simulink model "Model_Simulation"  (R2016a)
settings: Solver=FixedStepAuto  StartTime=0.0  StopTime=5  FixedStep=2e-6  RelTol=1e-3
values from neighbouring files (symbols this model uses):
  C = 3060e-6    (= 0.00306)    [Controle_Inversor_UR_D.m]
  Ki_i_disc = wc*Rf    (= 44.2477838534)    [Controle_Inversor_UR_D.m]
  Ki_i_disc_b = wc_b*Rb/Vdc    (= 0.0983284085631)    [Controle_Inversor_UR_D.m]
  Ki_q_disc = wq/H    [Controle_Inversor_UR_D.m]
  Ki_v_disc_b = wc_bv/Req    (= 14.5799013102)    [Controle_Inversor_UR_D.m]
  Ki_vdc_disc = ((wvdc)^2*C)/Gt    [Controle_Inversor_UR_D.m]
  Kp_i_disc = wc*Lf    (= 2.19688771906)    [Controle_Inversor_UR_D.m]
  Kp_i_disc_b = wc_b*Lb/Vdc    (= 0.00545604673435)    [Controle_Inversor_UR_D.m]
  Kp_q_disc = Ki_q_disc*(Lf/Kp_i_disc)    [Controle_Inversor_UR_D.m]
  Kp_v_disc_b = wc_bv*Cin    (= 0.0356301510224)    [Controle_Inversor_UR_D.m]
  Kp_vdc_disc = (2*ksi_vdc*wvdc*C)/Gt    [Controle_Inversor_UR_D.m]
  Lf = (0.0012+2.8949e-04)    (= 0.00148949)    [Controle_Inversor_UR_D.m]
  Tsw = 1/fsw    (= 0.0002)    [Controle_Inversor_UR_D.m]
  w = 2*pi*60    (= 376.991118431)    [Controle_Inversor_UR_D.m]
undefined symbols (not defined in the file or in its folder): D1, dEgdT, Delta, EgRef, gcbh, k1, Rsh_array5pc, sigbuilder_block, sps_rtmsupport, Tref_K, VT_ref
libraries: powerlib x179, simulink x14, powerlib_meascontrol x13, spsPVarrayModel x12
(part 19 of 20)

== system Model_Simulation/Subsystem2/DDSRF-PLL  ==
  Vabc : Inport
  Constant : Constant  Value=2*pi*60
  Demux : Demux  Outputs=3
  Função transferência LPF Fc = 42 Hz{,1..3} (4 alike) : TransferFcn  Numerator=[0 0 263.8937]  Denominator=[0 1 263.8937]
  Integrator : Integrator
  PID Controller : simulink/Continuous/PID Controller  Controller=PI  TimeDomain=Continuous-time  SampleTime=-1  IntegratorMethod=Forward Euler  FilterMethod=Forward Euler  Form=Parallel  UseFilter=on  ControllerParametersSource=internal  P=0.34  I=38.3  D=0  N=100  InitialConditionSource=internal  InitialConditionForIntegrator=0  InitialConditionForFilter=0  ExternalReset=none  LimitOutput=off  UpperSaturationLimit=inf  LowerSaturationLimit=-inf  LinearizeAsGain=on  AntiWindupMode=none  Kb=1  TrackingMode=off  Kt=1  PParamMin=[]  PParamMax=[]  IParamMin=[]  IParamMax=[]  DParamMin=[]  DParamMax=[]  NParamMin=[]  NParamMax=[]  KbParamMin=[]  KbParamMax=[]  KtParamMin=[]  KtParamMax=[]  POutMin=[]  POutMax=[]  IOutMin=[]  IOutMax=[]  DOutMin=[]  DOutMax=[]  NOutMin=[]  NOutMax=[]  KbOutMin=[]  KbOutMax=[]  KtOutMin=[]  KtOutMax=[]  IntegratorOutMin=[]  IntegratorOutMax=[]  FilterOutMin=[]  FilterOutMax=[]  SumOutMin=[]  SumOutMax=[]  SumI1OutMin=[]  SumI1OutMax=[]  SumI2OutMin=[]  SumI2OutMax=[]  SumI3OutMin=[]  SumI3OutMax=[]  SumDOutMin=[]  SumDOutMax=[]  SaturationOutMin=[]  SaturationOutMax=[]  IntegratorContinuousStateAttributes=''  IntegratorStateMustResolveToSignalObject=off  IntegratorRTWStateStorageClass=Auto  FilterContinuousStateAttributes=''  FilterStateMustResolveToSignalObject=off  FilterRTWStateStorageClass=Auto  DifferentiatorICPrevScaledInput=0  DifferentiatorOutMin=[]  DifferentiatorOutMax=[]
  Subsystem : Subsystem
  Subsystem1 : Subsystem
  Subsystem2 : Subsystem
  Subsystem3 : Subsystem
  Sum : Sum  Inputs=|++
  abc to Alpha-Beta-Zero1 : powerlib_meascontrol/Transformations/abc to Alpha-Beta-Zero
  wt : Outport
  wires:
  Vabc/1 -> abc to Alpha-Beta-Zero1/1
  abc to Alpha-Beta-Zero1/1 -> Demux/1
  Demux/1 -> Subsystem1/2(Alpha), Subsystem/2(Alpha)
  Demux/2 -> Subsystem1/3(Beta), Subsystem/3(Beta)
  Subsystem/1(Vd+) -> Subsystem2/1(Vd+)
  Subsystem/2(Vq+) -> Subsystem2/2(Vq+)
  Subsystem1/1(Vd-) -> Subsystem3/1(Vd-)
  Subsystem1/2(Vq-) -> Subsystem3/2(Vq-)
  Subsystem2/1(Vd*+) -> Função transferência LPF Fc = 42 Hz/1
  Subsystem3/1(Vd*-) -> Função transferência LPF Fc = 42 Hz2/1
  Subsystem3/2(Vq*-) -> Função transferência LPF Fc = 42 Hz3/1
  Função transferência LPF Fc = 42 Hz2/1 -> Subsystem2/3(Vd-)
  Função transferência LPF Fc = 42 Hz3/1 -> Subsystem2/4(Vq-)
  Subsystem2/2(Vq*+) -> PID Controller/1, Função transferência LPF Fc = 42 Hz1/1
  PID Controller/1 -> Sum/1
  Constant/1 -> Sum/2
  Sum/1 -> Integrator/1
  Integrator/1 -> Subsystem2/5(fase), Subsystem3/5(fase), Subsystem1/1(Fase), Subsystem/1(Fase), wt/1
  Função transferência LPF Fc = 42 Hz1/1 -> Subsystem3/4(Vq+)
  Função transferência LPF Fc = 42 Hz/1 -> Subsystem3/3(Vd+)

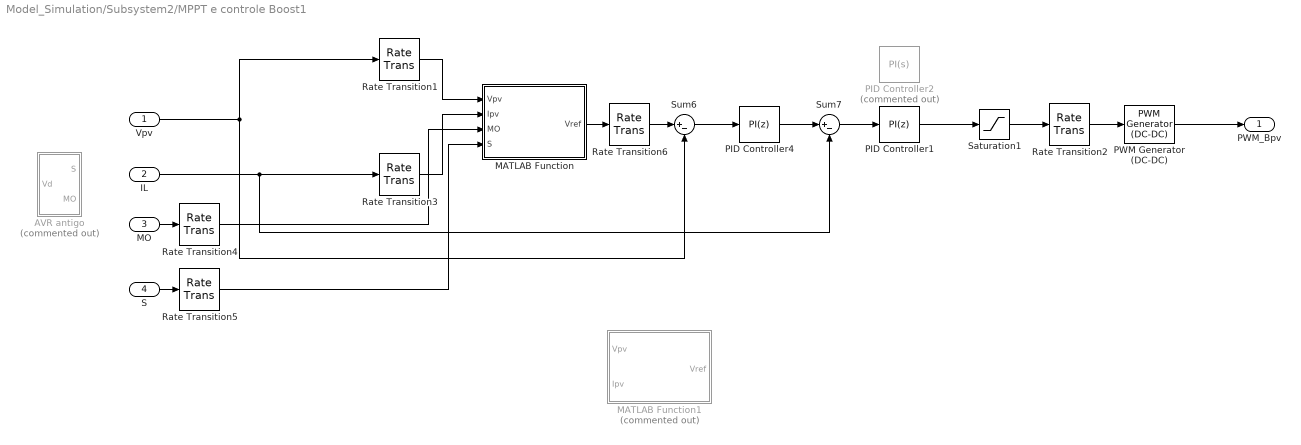
== system Model_Simulation/Subsystem2/MPPT e controle Boost1 ==
  Vpv : Inport
  IL : Inport  Port=2
  MO : Inport  Port=3
  S : Inport  Port=4
  AVR antigo : Subsystem  Commented=on
  MATLAB Function : MATLAB Function  TreatAsAtomicUnit=on
  MATLAB Function1 : MATLAB Function  Commented=on  TreatAsAtomicUnit=on
  PID Controller1 : simulink/Continuous/PID Controller  Controller=PI  TimeDomain=Discrete-time  SampleTime=-1  IntegratorMethod=Trapezoidal  FilterMethod=Forward Euler  Form=Parallel  UseFilter=on  ControllerParametersSource=internal  P=Kp_i_disc_b  I=Ki_i_disc_b  D=0  N=100  InitialConditionSource=internal  InitialConditionForIntegrator=0  InitialConditionForFilter=0  ExternalReset=none  LimitOutput=off  UpperSaturationLimit=inf  LowerSaturationLimit=-inf  LinearizeAsGain=on  AntiWindupMode=none  Kb=1  TrackingMode=off  Kt=1  PParamMin=[]  PParamMax=[]  IParamMin=[]  IParamMax=[]  DParamMin=[]  DParamMax=[]  NParamMin=[]  NParamMax=[]  KbParamMin=[]  KbParamMax=[]  KtParamMin=[]  KtParamMax=[]  POutMin=[]  POutMax=[]  IOutMin=[]  IOutMax=[]  DOutMin=[]  DOutMax=[]  NOutMin=[]  NOutMax=[]  KbOutMin=[]  KbOutMax=[]  KtOutMin=[]  KtOutMax=[]  IntegratorOutMin=[]  IntegratorOutMax=[]  FilterOutMin=[]  FilterOutMax=[]  SumOutMin=[]  SumOutMax=[]  SumI1OutMin=[]  SumI1OutMax=[]  SumI2OutMin=[]  SumI2OutMax=[]  SumI3OutMin=[]  SumI3OutMax=[]  SumDOutMin=[]  SumDOutMax=[]  SaturationOutMin=[]  SaturationOutMax=[]  IntegratorContinuousStateAttributes=''  IntegratorStateMustResolveToSignalObject=off  IntegratorRTWStateStorageClass=Auto  FilterContinuousStateAttributes=''  FilterStateMustResolveToSignalObject=off  FilterRTWStateStorageClass=Auto  DifferentiatorICPrevScaledInput=0  DifferentiatorOutMin=[]  DifferentiatorOutMax=[]
  PID Controller2 : simulink/Continuous/PID Controller  Commented=on  Controller=PI  TimeDomain=Continuous-time  SampleTime=-1  IntegratorMethod=Forward Euler  FilterMethod=Forward Euler  Form=Parallel  UseFilter=on  ControllerParametersSource=internal  P=0.00831222  I=15.393  D=0  N=100  InitialConditionSource=internal  InitialConditionForIntegrator=0  InitialConditionForFilter=0  ExternalReset=none  LimitOutput=off  UpperSaturationLimit=inf  LowerSaturationLimit=-inf  LinearizeAsGain=on  AntiWindupMode=none  Kb=1  TrackingMode=off  Kt=1  PParamMin=[]  PParamMax=[]  IParamMin=[]  IParamMax=[]  DParamMin=[]  DParamMax=[]  NParamMin=[]  NParamMax=[]  KbParamMin=[]  KbParamMax=[]  KtParamMin=[]  KtParamMax=[]  POutMin=[]  POutMax=[]  IOutMin=[]  IOutMax=[]  DOutMin=[]  DOutMax=[]  NOutMin=[]  NOutMax=[]  KbOutMin=[]  KbOutMax=[]  KtOutMin=[]  KtOutMax=[]  IntegratorOutMin=[]  IntegratorOutMax=[]  FilterOutMin=[]  FilterOutMax=[]  SumOutMin=[]  SumOutMax=[]  SumI1OutMin=[]  SumI1OutMax=[]  SumI2OutMin=[]  SumI2OutMax=[]  SumI3OutMin=[]  SumI3OutMax=[]  SumDOutMin=[]  SumDOutMax=[]  SaturationOutMin=[]  SaturationOutMax=[]  IntegratorContinuousStateAttributes=''  IntegratorStateMustResolveToSignalObject=off  IntegratorRTWStateStorageClass=Auto  FilterContinuousStateAttributes=''  FilterStateMustResolveToSignalObject=off  FilterRTWStateStorageClass=Auto  DifferentiatorICPrevScaledInput=0  DifferentiatorOutMin=[]  DifferentiatorOutMax=[]
  PID Controller4 : simulink/Continuous/PID Controller  Controller=PI  TimeDomain=Discrete-time  SampleTime=-1  IntegratorMethod=Trapezoidal  FilterMethod=Forward Euler  Form=Parallel  UseFilter=on  ControllerParametersSource=internal  P=-Kp_v_disc_b  I=-Ki_v_disc_b  D=0  N=100  InitialConditionSource=internal  InitialConditionForIntegrator=0  InitialConditionForFilter=0  ExternalReset=none  LimitOutput=off  UpperSaturationLimit=inf  LowerSaturationLimit=-inf  LinearizeAsGain=on  AntiWindupMode=none  Kb=1  TrackingMode=off  Kt=1  PParamMin=[]  PParamMax=[]  IParamMin=[]  IParamMax=[]  DParamMin=[]  DParamMax=[]  NParamMin=[]  NParamMax=[]  KbParamMin=[]  KbParamMax=[]  KtParamMin=[]  KtParamMax=[]  POutMin=[]  POutMax=[]  IOutMin=[]  IOutMax=[]  DOutMin=[]  DOutMax=[]  NOutMin=[]  NOutMax=[]  KbOutMin=[]  KbOutMax=[]  KtOutMin=[]  KtOutMax=[]  IntegratorOutMin=[]  IntegratorOutMax=[]  FilterOutMin=[]  FilterOutMax=[]  SumOutMin=[]  SumOutMax=[]  SumI1OutMin=[]  SumI1OutMax=[]  SumI2OutMin=[]  SumI2OutMax=[]  SumI3OutMin=[]  SumI3OutMax=[]  SumDOutMin=[]  SumDOutMax=[]  SaturationOutMin=[]  SaturationOutMax=[]  IntegratorContinuousStateAttributes=''  IntegratorStateMustResolveToSignalObject=off  IntegratorRTWStateStorageClass=Auto  FilterContinuousStateAttributes=''  FilterStateMustResolveToSignalObject=off  FilterRTWStateStorageClass=Auto  DifferentiatorICPrevScaledInput=0  DifferentiatorOutMin=[]  DifferentiatorOutMax=[]
  PWM Generator (DC-DC) : powerlib_meascontrol/Pulse & Signal Generators/PWM Generator (DC-DC)  Fsw=5e3  Ts=2e-6
  Rate Transition{1,3..5} (4 alike) : RateTransition  OutPortSampleTime=0.01
  Rate Transition2 : RateTransition  OutPortSampleTime=2e-6
  Rate Transition6 : RateTransition  OutPortSampleTime=Tsw
  Saturation1 : Saturate  UpperLimit=1  LowerLimit=0.01
  Sum6 : Sum  Inputs=|+-
  Sum7 : Sum  Inputs=|+-
  PWM_Bpv : Outport
  wires:
  PID Controller4/1 -> Sum7/1
  Sum6/1 -> PID Controller4/1
  PWM Generator (DC-DC)/1 -> PWM_Bpv/1
  Sum7/1 -> PID Controller1/1
  PID Controller1/1 -> Saturation1/1
  Saturation1/1 -> Rate Transition2/1
  MATLAB Function/1(Vref) -> Rate Transition6/1
  Vpv/1 -> Rate Transition1/1, Sum6/2
  IL/1 -> Rate Transition3/1, Sum7/2
  MO/1 -> Rate Transition4/1
  S/1 -> Rate Transition5/1
  Rate Transition2/1 -> PWM Generator (DC-DC)/1
  Rate Transition1/1 -> MATLAB Function/1(Vpv)
  Rate Transition3/1 -> MATLAB Function/2(Ipv)
  Rate Transition4/1 -> MATLAB Function/3(MO)
  Rate Transition5/1 -> MATLAB Function/4(S)
  Rate Transition6/1 -> Sum6/1

== system Model_Simulation/Subsystem2/MPPT e controle Boost2 ==
  Vpv : Inport
  IL : Inport  Port=2
  MO : Inport  Port=3
  S : Inport  Port=4
  MATLAB Function : MATLAB Function  TreatAsAtomicUnit=on
  MATLAB Function1 : MATLAB Function  Commented=on  TreatAsAtomicUnit=on
  PID Controller1 : simulink/Continuous/PID Controller  Controller=PI  TimeDomain=Discrete-time  SampleTime=-1  IntegratorMethod=Trapezoidal  FilterMethod=Forward Euler  Form=Parallel  UseFilter=on  ControllerParametersSource=internal  P=Kp_i_disc_b  I=Ki_i_disc_b  D=0  N=100  InitialConditionSource=internal  InitialConditionForIntegrator=0  InitialConditionForFilter=0  ExternalReset=none  LimitOutput=off  UpperSaturationLimit=inf  LowerSaturationLimit=-inf  LinearizeAsGain=on  AntiWindupMode=none  Kb=1  TrackingMode=off  Kt=1  PParamMin=[]  PParamMax=[]  IParamMin=[]  IParamMax=[]  DParamMin=[]  DParamMax=[]  NParamMin=[]  NParamMax=[]  KbParamMin=[]  KbParamMax=[]  KtParamMin=[]  KtParamMax=[]  POutMin=[]  POutMax=[]  IOutMin=[]  IOutMax=[]  DOutMin=[]  DOutMax=[]  NOutMin=[]  NOutMax=[]  KbOutMin=[]  KbOutMax=[]  KtOutMin=[]  KtOutMax=[]  IntegratorOutMin=[]  IntegratorOutMax=[]  FilterOutMin=[]  FilterOutMax=[]  SumOutMin=[]  SumOutMax=[]  SumI1OutMin=[]  SumI1OutMax=[]  SumI2OutMin=[]  SumI2OutMax=[]  SumI3OutMin=[]  SumI3OutMax=[]  SumDOutMin=[]  SumDOutMax=[]  SaturationOutMin=[]  SaturationOutMax=[]  IntegratorContinuousStateAttributes=''  IntegratorStateMustResolveToSignalObject=off  IntegratorRTWStateStorageClass=Auto  FilterContinuousStateAttributes=''  FilterStateMustResolveToSignalObject=off  FilterRTWStateStorageClass=Auto  DifferentiatorICPrevScaledInput=0  DifferentiatorOutMin=[]  DifferentiatorOutMax=[]
  PID Controller2 : simulink/Continuous/PID Controller  Commented=on  Controller=PI  TimeDomain=Continuous-time  SampleTime=-1  IntegratorMethod=Forward Euler  FilterMethod=Forward Euler  Form=Parallel  UseFilter=on  ControllerParametersSource=internal  P=-0.02947505  I=-5.3591  D=0  N=100  InitialConditionSource=internal  InitialConditionForIntegrator=0  InitialConditionForFilter=0  ExternalReset=none  LimitOutput=off  UpperSaturationLimit=inf  LowerSaturationLimit=-inf  LinearizeAsGain=on  AntiWindupMode=none  Kb=1  TrackingMode=off  Kt=1  PParamMin=[]  PParamMax=[]  IParamMin=[]  IParamMax=[]  DParamMin=[]  DParamMax=[]  NParamMin=[]  NParamMax=[]  KbParamMin=[]  KbParamMax=[]  KtParamMin=[]  KtParamMax=[]  POutMin=[]  POutMax=[]  IOutMin=[]  IOutMax=[]  DOutMin=[]  DOutMax=[]  NOutMin=[]  NOutMax=[]  KbOutMin=[]  KbOutMax=[]  KtOutMin=[]  KtOutMax=[]  IntegratorOutMin=[]  IntegratorOutMax=[]  FilterOutMin=[]  FilterOutMax=[]  SumOutMin=[]  SumOutMax=[]  SumI1OutMin=[]  SumI1OutMax=[]  SumI2OutMin=[]  SumI2OutMax=[]  SumI3OutMin=[]  SumI3OutMax=[]  SumDOutMin=[]  SumDOutMax=[]  SaturationOutMin=[]  SaturationOutMax=[]  IntegratorContinuousStateAttributes=''  IntegratorStateMustResolveToSignalObject=off  IntegratorRTWStateStorageClass=Auto  FilterContinuousStateAttributes=''  FilterStateMustResolveToSignalObject=off  FilterRTWStateStorageClass=Auto  DifferentiatorICPrevScaledInput=0  DifferentiatorOutMin=[]  DifferentiatorOutMax=[]
  PID Controller4 : simulink/Continuous/PID Controller  Controller=PI  TimeDomain=Discrete-time  SampleTime=-1  IntegratorMethod=Trapezoidal  FilterMethod=Forward Euler  Form=Parallel  UseFilter=on  ControllerParametersSource=internal  P=-Kp_v_disc_b  I=-Ki_v_disc_b  D=0  N=100  InitialConditionSource=internal  InitialConditionForIntegrator=0  InitialConditionForFilter=0  ExternalReset=none  LimitOutput=off  UpperSaturationLimit=inf  LowerSaturationLimit=-inf  LinearizeAsGain=on  AntiWindupMode=none  Kb=1  TrackingMode=off  Kt=1  PParamMin=[]  PParamMax=[]  IParamMin=[]  IParamMax=[]  DParamMin=[]  DParamMax=[]  NParamMin=[]  NParamMax=[]  KbParamMin=[]  KbParamMax=[]  KtParamMin=[]  KtParamMax=[]  POutMin=[]  POutMax=[]  IOutMin=[]  IOutMax=[]  DOutMin=[]  DOutMax=[]  NOutMin=[]  NOutMax=[]  KbOutMin=[]  KbOutMax=[]  KtOutMin=[]  KtOutMax=[]  IntegratorOutMin=[]  IntegratorOutMax=[]  FilterOutMin=[]  FilterOutMax=[]  SumOutMin=[]  SumOutMax=[]  SumI1OutMin=[]  SumI1OutMax=[]  SumI2OutMin=[]  SumI2OutMax=[]  SumI3OutMin=[]  SumI3OutMax=[]  SumDOutMin=[]  SumDOutMax=[]  SaturationOutMin=[]  SaturationOutMax=[]  IntegratorContinuousStateAttributes=''  IntegratorStateMustResolveToSignalObject=off  IntegratorRTWStateStorageClass=Auto  FilterContinuousStateAttributes=''  FilterStateMustResolveToSignalObject=off  FilterRTWStateStorageClass=Auto  DifferentiatorICPrevScaledInput=0  DifferentiatorOutMin=[]  DifferentiatorOutMax=[]
  PWM Generator (DC-DC) : powerlib_meascontrol/Pulse & Signal Generators/PWM Generator (DC-DC)  Fsw=5e3  Ts=2e-6
  Rate Transition{1,3..5} (4 alike) : RateTransition  OutPortSampleTime=0.01
  Rate Transition2 : RateTransition  OutPortSampleTime=2e-6
  Rate Transition6 : RateTransition  OutPortSampleTime=Tsw
  Saturation1 : Saturate  UpperLimit=1  LowerLimit=0.01
  Sum6 : Sum  Inputs=|+-
  Sum7 : Sum  Inputs=|+-
  PWM_Bpv : Outport
  wires:
  IL/1 -> Rate Transition3/1, Sum7/2
  Vpv/1 -> Rate Transition1/1, Sum6/2
  MATLAB Function/1(Vref) -> Rate Transition6/1
  Saturation1/1 -> Rate Transition2/1
  PID Controller1/1 -> Saturation1/1
  Sum7/1 -> PID Controller1/1
  PWM Generator (DC-DC)/1 -> PWM_Bpv/1
  Sum6/1 -> PID Controller4/1
  PID Controller4/1 -> Sum7/1
  MO/1 -> Rate Transition5/1
  S/1 -> Rate Transition4/1
  Rate Transition2/1 -> PWM Generator (DC-DC)/1
  Rate Transition1/1 -> MATLAB Function/1(Vpv)
  Rate Transition3/1 -> MATLAB Function/2(Ipv)
  Rate Transition4/1 -> MATLAB Function/4(S)
  Rate Transition5/1 -> MATLAB Function/3(MO)
  Rate Transition6/1 -> Sum6/1

== system Model_Simulation/Subsystem2/MPPT e controle Boost3 ==
  Vpv : Inport
  IL : Inport  Port=2
  MO : Inport  Port=3
  S : Inport  Port=4
  MATLAB Function : MATLAB Function  TreatAsAtomicUnit=on
  PID Controller1 : simulink/Continuous/PID Controller  Controller=PI  TimeDomain=Discrete-time  SampleTime=-1  IntegratorMethod=Trapezoidal  FilterMethod=Forward Euler  Form=Parallel  UseFilter=on  ControllerParametersSource=internal  P=Kp_i_disc_b  I=Ki_i_disc_b  D=0  N=100  InitialConditionSource=internal  InitialConditionForIntegrator=0  InitialConditionForFilter=0  ExternalReset=none  LimitOutput=off  UpperSaturationLimit=inf  LowerSaturationLimit=-inf  LinearizeAsGain=on  AntiWindupMode=none  Kb=1  TrackingMode=off  Kt=1  PParamMin=[]  PParamMax=[]  IParamMin=[]  IParamMax=[]  DParamMin=[]  DParamMax=[]  NParamMin=[]  NParamMax=[]  KbParamMin=[]  KbParamMax=[]  KtParamMin=[]  KtParamMax=[]  POutMin=[]  POutMax=[]  IOutMin=[]  IOutMax=[]  DOutMin=[]  DOutMax=[]  NOutMin=[]  NOutMax=[]  KbOutMin=[]  KbOutMax=[]  KtOutMin=[]  KtOutMax=[]  IntegratorOutMin=[]  IntegratorOutMax=[]  FilterOutMin=[]  FilterOutMax=[]  SumOutMin=[]  SumOutMax=[]  SumI1OutMin=[]  SumI1OutMax=[]  SumI2OutMin=[]  SumI2OutMax=[]  SumI3OutMin=[]  SumI3OutMax=[]  SumDOutMin=[]  SumDOutMax=[]  SaturationOutMin=[]  SaturationOutMax=[]  IntegratorContinuousStateAttributes=''  IntegratorStateMustResolveToSignalObject=off  IntegratorRTWStateStorageClass=Auto  FilterContinuousStateAttributes=''  FilterStateMustResolveToSignalObject=off  FilterRTWStateStorageClass=Auto  DifferentiatorICPrevScaledInput=0  DifferentiatorOutMin=[]  DifferentiatorOutMax=[]
  PID Controller4 : simulink/Continuous/PID Controller  Controller=PI  TimeDomain=Discrete-time  SampleTime=-1  IntegratorMethod=Trapezoidal  FilterMethod=Forward Euler  Form=Parallel  UseFilter=on  ControllerParametersSource=internal  P=-Kp_v_disc_b  I=-Ki_v_disc_b  D=0  N=100  InitialConditionSource=internal  InitialConditionForIntegrator=0  InitialConditionForFilter=0  ExternalReset=none  LimitOutput=off  UpperSaturationLimit=inf  LowerSaturationLimit=-inf  LinearizeAsGain=on  AntiWindupMode=none  Kb=1  TrackingMode=off  Kt=1  PParamMin=[]  PParamMax=[]  IParamMin=[]  IParamMax=[]  DParamMin=[]  DParamMax=[]  NParamMin=[]  NParamMax=[]  KbParamMin=[]  KbParamMax=[]  KtParamMin=[]  KtParamMax=[]  POutMin=[]  POutMax=[]  IOutMin=[]  IOutMax=[]  DOutMin=[]  DOutMax=[]  NOutMin=[]  NOutMax=[]  KbOutMin=[]  KbOutMax=[]  KtOutMin=[]  KtOutMax=[]  IntegratorOutMin=[]  IntegratorOutMax=[]  FilterOutMin=[]  FilterOutMax=[]  SumOutMin=[]  SumOutMax=[]  SumI1OutMin=[]  SumI1OutMax=[]  SumI2OutMin=[]  SumI2OutMax=[]  SumI3OutMin=[]  SumI3OutMax=[]  SumDOutMin=[]  SumDOutMax=[]  SaturationOutMin=[]  SaturationOutMax=[]  IntegratorContinuousStateAttributes=''  IntegratorStateMustResolveToSignalObject=off  IntegratorRTWStateStorageClass=Auto  FilterContinuousStateAttributes=''  FilterStateMustResolveToSignalObject=off  FilterRTWStateStorageClass=Auto  DifferentiatorICPrevScaledInput=0  DifferentiatorOutMin=[]  DifferentiatorOutMax=[]
  PWM Generator (DC-DC) : powerlib_meascontrol/Pulse & Signal Generators/PWM Generator (DC-DC)  Fsw=5e3  Ts=2e-6
  Rate Transition{1,3..5} (4 alike) : RateTransition  OutPortSampleTime=0.01
  Rate Transition2 : RateTransition  OutPortSampleTime=2e-6
  Rate Transition6 : RateTransition  OutPortSampleTime=Tsw
  Saturation1 : Saturate  UpperLimit=1  LowerLimit=0.01
  Sum6 : Sum  Inputs=|+-
  Sum7 : Sum  Inputs=|+-
  PWM_Bpv : Outport
  wires:
  PID Controller4/1 -> Sum7/1
  Sum6/1 -> PID Controller4/1
  PWM Generator (DC-DC)/1 -> PWM_Bpv/1
  Sum7/1 -> PID Controller1/1
  PID Controller1/1 -> Saturation1/1
  Saturation1/1 -> Rate Transition2/1
  MATLAB Function/1(Vref) -> Rate Transition6/1
  Vpv/1 -> Rate Transition1/1, Sum6/2
  IL/1 -> Rate Transition3/1, Sum7/2
  MO/1 -> Rate Transition4/1
  S/1 -> Rate Transition5/1
  Rate Transition2/1 -> PWM Generator (DC-DC)/1
  Rate Transition1/1 -> MATLAB Function/1(Vpv)
  Rate Transition3/1 -> MATLAB Function/2(Ipv)
  Rate Transition4/1 -> MATLAB Function/3(MO)
  Rate Transition5/1 -> MATLAB Function/4(S)
  Rate Transition6/1 -> Sum6/1

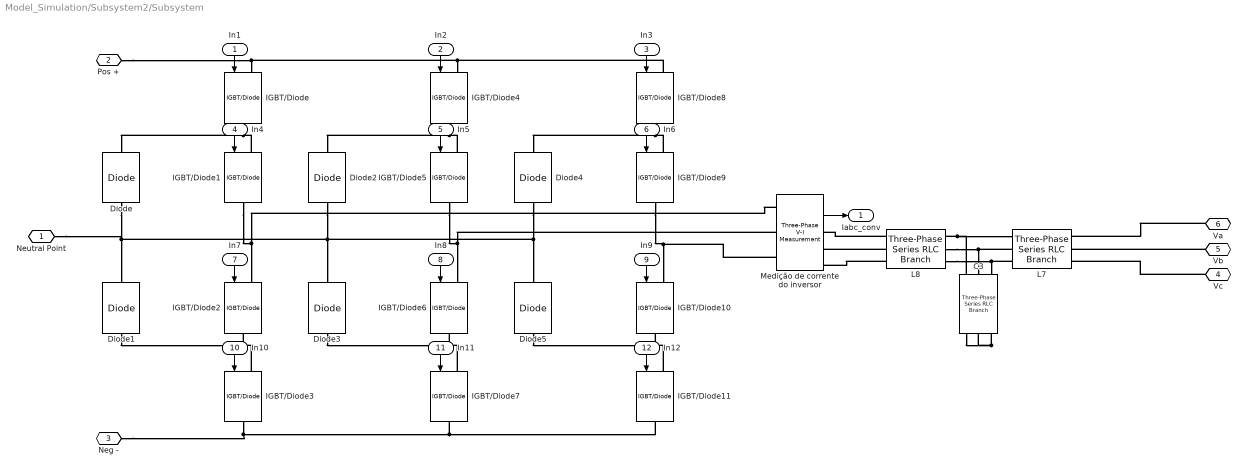
== system Model_Simulation/Subsystem2/Subsystem ==
  In1 : Inport
  In2 : Inport  Port=2
  In3 : Inport  Port=3
  In4 : Inport  Port=4
  In5 : Inport  Port=5
  In6 : Inport  Port=6
  In7 : Inport  Port=7
  In8 : Inport  Port=8
  In9 : Inport  Port=9
  In10 : Inport  Port=10
  In11 : Inport  Port=11
  In12 : Inport  Port=12
  C3 : powerlib/Elements/Three-Phase Series RLC Branch  LConnTagsString=A|B|C  RConnTagsString=A|B|C  BranchType=RC  Resistance=0.9228  Inductance=1e-3  Capacitance=3.4534e-05  Measurements=None
  Diode{,1..5} (6 alike) : powerlib/Power Electronics/Diode  Ron=0.001  Lon=0  Vf=0.8  IC=0  UseSnubber=off  Rs=500  Cs=250e-9  Measurements=off
  IGBT/Diode{,1..11} (12 alike) : powerlib/Power Electronics/IGBT//Diode  Ron=1e-3  Rs=1e5  Cs=inf  Measurements=off
  L7 : powerlib/Elements/Three-Phase Series RLC Branch  LConnTagsString=A|B|C  RConnTagsString=A|B|C  BranchType=RL  Resistance=0.015  Inductance=3.3006e-04  Capacitance=1e-6  Measurements=None
  L8 : powerlib/Elements/Three-Phase Series RLC Branch  LConnTagsString=A|B|C  RConnTagsString=A|B|C  BranchType=RL  Resistance=0.015  Inductance=0.0013  Capacitance=1e-6  Measurements=None
  Medição de corrente do inversor : powerlib/Measurements/Three-Phase V-I Measurement  VoltageMeasurement=phase-to-ground  SetLabelV=off  LabelV=Vabc  Vpu=off  VpuLL=off  CurrentMeasurement=yes  SetLabelI=off  LabelI=Iabc  Ipu=off  Pbase=100e6  Vbase=500e3  OutputType=Complex  PhasorSimulation=off  PSBequivalent=0
  Neutral Point : PMIOPort  Port=1  Side=Left
  Pos + : PMIOPort  Port=2  Side=Left
  Neg - : PMIOPort  Port=3  Side=Left
  Vc : PMIOPort  Port=4  Side=Right
  Vb : PMIOPort  Port=5  Side=Right
  Va : PMIOPort  Port=6  Side=Right
  Iabc_conv : Outport
  wires:
  In10/1 -> IGBT/Diode3/1
  In8/1 -> IGBT/Diode6/1
  In7/1 -> IGBT/Diode2/1
  In9/1 -> IGBT/Diode10/1
  In6/1 -> IGBT/Diode9/1
  In12/1 -> IGBT/Diode11/1
  In4/1 -> IGBT/Diode1/1
  In1/1 -> IGBT/Diode/1
  In3/1 -> IGBT/Diode8/1
  In2/1 -> IGBT/Diode4/1
  In11/1 -> IGBT/Diode7/1
  In5/1 -> IGBT/Diode5/1
  Medição de corrente do inversor/2 -> Iabc_conv/1
  connections:
  IGBT/Diode1/LConn1 -- Diode/RConn1 -- IGBT/Diode/RConn1
  IGBT/Diode3/RConn1 -- Neg -/RConn1 -- IGBT/Diode11/RConn1 -- IGBT/Diode7/RConn1
  IGBT/Diode11/LConn1 -- Diode5/LConn1 -- IGBT/Diode10/RConn1
  IGBT/Diode9/RConn1 -- Medição de corrente do inversor/LConn3 -- IGBT/Diode10/LConn1
  IGBT/Diode8/RConn1 -- IGBT/Diode9/LConn1 -- Diode4/RConn1
  IGBT/Diode3/LConn1 -- Diode1/LConn1 -- IGBT/Diode2/RConn1
  IGBT/Diode8/LConn1 -- Pos +/RConn1 -- IGBT/Diode/LConn1 -- IGBT/Diode4/LConn1
  IGBT/Diode5/RConn1 -- IGBT/Diode6/LConn1 -- Medição de corrente do inversor/LConn2
  Diode4/LConn1 -- Diode2/LConn1 -- Neutral Point/RConn1 -- Diode/LConn1 -- Diode1/RConn1 -- Diode3/RConn1 -- Diode5/RConn1
  Diode3/LConn1 -- IGBT/Diode7/LConn1 -- IGBT/Diode6/RConn1
  IGBT/Diode5/LConn1 -- IGBT/Diode4/RConn1 -- Diode2/RConn1
  IGBT/Diode1/RConn1 -- IGBT/Diode2/LConn1 -- Medição de corrente do inversor/LConn1
  L8/RConn2 -- C3/LConn2 -- L7/LConn2
  L8/RConn3 -- C3/LConn3 -- L7/LConn3
  C3/RConn3 -- C3/RConn2 -- C3/RConn1
  L8/RConn1 -- C3/LConn1 -- L7/LConn1
  Va/RConn1 -- L7/RConn1
  Vc/RConn1 -- L7/RConn3
  L8/LConn1 -- Medição de corrente do inversor/RConn1
  L8/LConn2 -- Medição de corrente do inversor/RConn2
  L8/LConn3 -- Medição de corrente do inversor/RConn3
  Vb/RConn1 -- L7/RConn2

== system Model_Simulation/Subsystem2/Subsystem1 ==
  PWM : Inport
  C3 : powerlib/Elements/Three-Phase Series RLC Branch  LConnTagsString=A|B|C  RConnTagsString=A|B|C  BranchType=RC  Resistance=0.8094  Inductance=1e-3  Capacitance=3.9374e-05  Measurements=None
  L7 : powerlib/Elements/Three-Phase Series RLC Branch  LConnTagsString=A|B|C  RConnTagsString=A|B|C  BranchType=RL  Resistance=0.015  Inductance=2.8949e-04  Capacitance=1e-6  Measurements=None
  L8 : powerlib/Elements/Three-Phase Series RLC Branch  LConnTagsString=A|B|C  RConnTagsString=A|B|C  BranchType=RL  Resistance=0.015  Inductance=0.0012  Capacitance=1e-6  Measurements=None
  Medição de corrente do inversor : powerlib/Measurements/Three-Phase V-I Measurement  VoltageMeasurement=no  SetLabelV=off  LabelV=Vabc  Vpu=off  VpuLL=off  CurrentMeasurement=yes  SetLabelI=off  LabelI=Iabc  Ipu=off  Pbase=100e6  Vbase=500e3  OutputType=Complex  PhasorSimulation=off  PSBequivalent=0
  Three-Level NPC Converter : powerlib/Power Electronics/Three-Level NPC Converter  ModelType=Switching devices  Ron=1e-3  Rs=1e6  Cs=inf  Vforward=[0,0]  Ron_Diode=1e-3  Rs_Diode=1e6  Cs_Diode=inf  Vf_Diode=1e-3  Rs_CurrentSource=inf
  Vdc : powerlib/Measurements/Voltage Measurement  PhasorSimulation=off  OutputType=Complex  PSBequivalent=0
  Pos + : PMIOPort  Port=1  Side=Left
  Neutral Point : PMIOPort  Port=2  Side=Left
  Neg - : PMIOPort  Port=3  Side=Left
  Va : PMIOPort  Port=4  Side=Right
  Vb : PMIOPort  Port=5  Side=Right
  Vc : PMIOPort  Port=6  Side=Right
  Iabc_conv : Outport
  V_dc : Outport  Port=2
  wires:
  Medição de corrente do inversor/1 -> Iabc_conv/1
  Vdc/1 -> V_dc/1
  PWM/1 -> Three-Level NPC Converter/1
  connections:
  Vb/RConn1 -- L7/RConn2
  L8/LConn3 -- Medição de corrente do inversor/RConn3
  L8/LConn2 -- Medição de corrente do inversor/RConn2
  L8/LConn1 -- Medição de corrente do inversor/RConn1
  Vc/RConn1 -- L7/RConn3
  Va/RConn1 -- L7/RConn1
  C3/LConn1 -- L8/RConn1 -- L7/LConn1
  C3/RConn2 -- C3/RConn3 -- C3/RConn1
  C3/LConn3 -- L8/RConn3 -- L7/LConn3
  C3/LConn2 -- L8/RConn2 -- L7/LConn2
  Medição de corrente do inversor/LConn2 -- Three-Level NPC Converter/LConn2
  Medição de corrente do inversor/LConn1 -- Three-Level NPC Converter/LConn1
  Medição de corrente do inversor/LConn3 -- Three-Level NPC Converter/LConn3
  Pos +/RConn1 -- Vdc/LConn1 -- Three-Level NPC Converter/RConn1
  Neg -/RConn1 -- Vdc/LConn2 -- Three-Level NPC Converter/RConn3
  Neutral Point/RConn1 -- Three-Level NPC Converter/RConn2

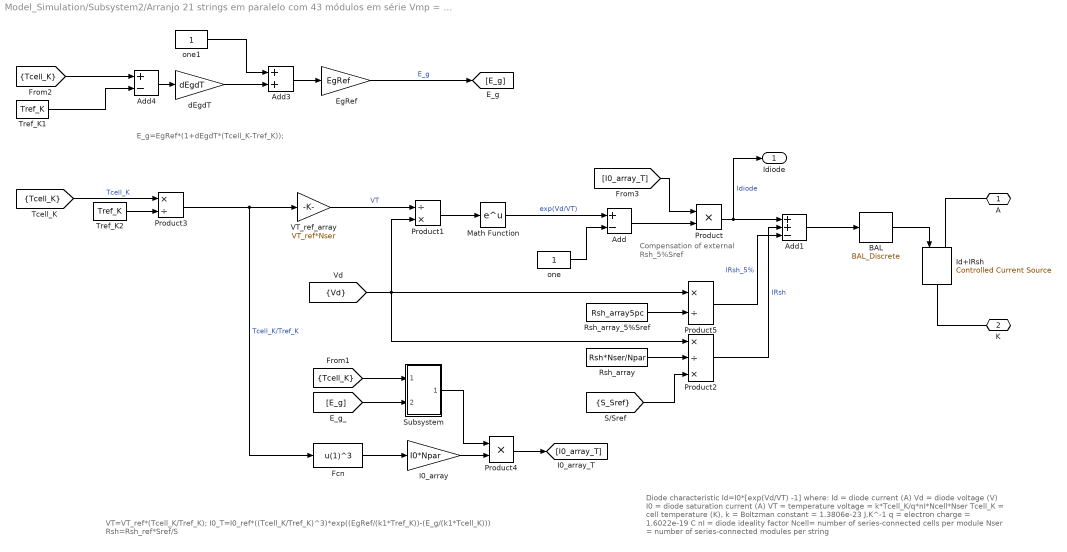
== system Model_Simulation/Subsystem2/Arranjo 21 strings em paralelo com 43 módulos em série Vmp = 43 x 30,6 = 1315,8 V Imp = 8,32 x 21 = 174,72 A 229.896,576 W/Diode Rsh ==
  note: E_g=EgRef*(1+dEgdT*(Tcell_K-Tref_K));
  note: VT=VT_ref*(Tcell_K/Tref_K);
      | I0_T=I0_ref*((Tcell_K/Tref_K)^3)*exp((EgRef/(k1*Tref_K))-(E_g/(k1*Tcell_K)))
      | Rsh=Rsh_ref*Sref/S
  note: Diode characteristic
      |    Id=I0*[exp(Vd/VT) -1]
      |
      | where:
      |      Id = diode current (A)
      |      Vd = diode voltage (V)
      |      I0 = diode saturation current (A)
      |      VT = temperature voltage = k*Tcell_K/q*nI*Ncell*Nser
      | Tcell_K = cell temperature (K),
      |       k = Boltzman constant = 1.3806e-23 J.K^-1
      |       q = electron charge = 1.6022e-19 C
      |      nI = diode ideality factor
      |    Ncell= number of series-connected cells per module
      |    Nser = number of series-connected modules per string
  note: Compensation of
      | external Rsh_5%Sref
  Add : Sum  Inputs=+-
  Add1 : Sum  Inputs=++-
  Add3 : Sum
  Add4 : Sum  Inputs=+-
  BAL : spsPVarrayModel/BAL_Discrete  VariantControl=NoBAL
  EgRef : Gain  Gain=EgRef
  Fcn : Fcn  Expr=u(1)^3
  I0_array : Gain  Gain=I0*Npar
  Id+IRsh : powerlib/Electrical Sources/Controlled Current Source  Initialize=on  Source_Type=AC  Amplitude=0  Phase=0  Frequency=0  Measurements=None
  Math Function : Math  SaturateOnIntegerOverflow=on
  Product : Product  RndMeth=Zero
  Product1 : Product  Inputs=/*  RndMeth=Zero
  Product2 : Product  Inputs=*/*  RndMeth=Zero
  Product3 : Product  Inputs=*/  RndMeth=Zero
  Product4 : Product  Inputs=**  RndMeth=Zero
  Product5 : Product  Inputs=*/  RndMeth=Zero
  Rsh_array : Constant  Value=Rsh*Nser/Npar
  Rsh_array_5%Sref : Constant  Value=Rsh_array5pc
  Subsystem : Subsystem
  Tref_K1 : Constant  Value=Tref_K
  Tref_K2 : Constant  Value=Tref_K
  VT_ref_array : Gain  Gain=VT_ref*Nser
  dEgdT : Gain  Gain=dEgdT
  one : Constant
  one1 : Constant
  A : PMIOPort  Port=1  Side=Left
  K : PMIOPort  Port=2  Side=Right
  Idiode : Outport
  wires:
  [Vd] -> Product1/2, Product2/1, Product5/1
  [S_Sref] -> Product2/3
  [I0_array_T] -> Product/1
  VT_ref_array/1 -> Product1/1  "VT"
  Add/1 -> Product/2
  Product4/1 -> [I0_array_T]
  Tref_K2/1 -> Product3/2
  [E_g] -> Subsystem/2(E_g)
  [Tcell_K] -> Subsystem/1(Tcell_K)
  Subsystem/1(exp) -> Product4/1
  Tref_K1/1 -> Add4/2
  [Tcell_K] -> Add4/1
  Fcn/1 -> I0_array/1
  I0_array/1 -> Product4/2
  EgRef/1 -> [E_g]  "E_g"
  Add3/1 -> EgRef/1
  dEgdT/1 -> Add3/2
  Add4/1 -> dEgdT/1
  one1/1 -> Add3/1
  Product3/1 -> Fcn/1, VT_ref_array/1  "Tcell_K/Tref_K"
  [Tcell_K] -> Product3/1  "Tcell_K"
  Rsh_array/1 -> Product2/2
  one/1 -> Add/2
  Product1/1 -> Math Function/1
  Product/1 -> Idiode/1, Add1/1  "Idiode"
  Product2/1 -> Add1/2  "IRsh"
  Math Function/1 -> Add/1  "exp(Vd/VT)"
  Rsh_array_5%Sref/1 -> Product5/2
  Product5/1 -> Add1/3  "IRsh_5%"
  Add1/1 -> BAL/1
  BAL/1 -> Id+IRsh/1
  connections:
  A/RConn1 -- Id+IRsh/LConn1
  Id+IRsh/RConn1 -- K/RConn1

== system Model_Simulation/Subsystem2/Arranjo 21 strings em paralelo com 43 módulos em série Vmp = 43 x 30,6 = 1315,8 V Imp = 8,32 x 21 = 174,72 A 229.896,576 W/IL ctrl ==
  note: IL=S/Sref*(IL_ref+alpha_isc*(Tcell_K-Tref_K));
  Temperature : Inport
  Irradiance : Inport  Port=2
  0_K : Constant  Value=273.15
  1/Sref : Gain  Gain=1e-3
  Add : Sum
  Add2 : Sum
  Add3 : Sum  Inputs=+-
  IL_module : Constant  Value=IL
  Npar : Gain  Gain=Npar
  Product1 : Product  Inputs=**  RndMeth=Zero
  Tref_K : Constant  Value=Tref_K
  alpha_Isc : Gain  Gain=alpha_Isc
  IL : Outport
  tag scope: S_Sref=scoped, Tcell_K=scoped
  wires:
  1/Sref/1 -> [S_Sref], Product1/2  "S/Sref"
  Npar/1 -> Product1/1
  Add2/1 -> [Tcell_K], Add3/1  "Tcell_K"
  Add/1 -> Npar/1
  0_K/1 -> Add2/2
  IL_module/1 -> Add/2
  Product1/1 -> IL/1  "IL"
  Tref_K/1 -> Add3/2
  Add3/1 -> alpha_Isc/1
  alpha_Isc/1 -> Add/1
  Irradiance/1 -> 1/Sref/1
  Temperature/1 -> Add2/1

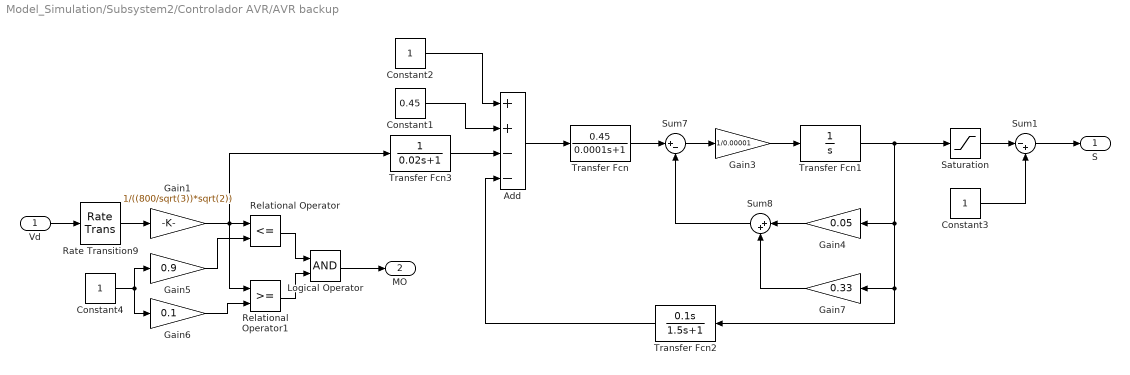
== system Model_Simulation/Subsystem2/Controlador AVR/AVR backup ==
  Vd : Inport
  Add : Sum  Inputs=++--
  Constant1 : Constant  Value=0.45
  Constant2 : Constant
  Constant3 : Constant
  Constant4 : Constant
  Gain1 : Gain  Gain=1/((800/sqrt(3))*sqrt(2))
  Gain3 : Gain  Gain=1/0.00001
  Gain4 : Gain  Gain=0.05
  Gain5 : Gain  Gain=0.9
  Gain6 : Gain  Gain=0.1
  Gain7 : Gain  Gain=0.33
  Logical Operator : Logic  AllPortsSameDT=off  OutDataTypeStr=boolean
  Rate Transition9 : RateTransition  OutPortSampleTime=2e-6
  Relational Operator : RelationalOperator  Operator=<=  OutDataTypeStr=boolean
  Relational Operator1 : RelationalOperator  OutDataTypeStr=boolean
  Saturation : Saturate  UpperLimit=1  LowerLimit=0
  Sum1 : Sum  Inputs=|-+
  Sum7 : Sum  Inputs=|+-
  Sum8 : Sum  Inputs=|++
  Transfer Fcn : TransferFcn  Numerator=[0.45]  Denominator=[0.0001 1]
  Transfer Fcn1 : TransferFcn  Denominator=[1 0]
  Transfer Fcn2 : TransferFcn  Numerator=[0.1 0]  Denominator=[1.5 1]
  Transfer Fcn3 : TransferFcn  Denominator=[0.02 1]
  S : Outport
  MO : Outport  Port=2
  wires:
  Constant3/1 -> Sum1/2
  Sum1/1 -> S/1
  Saturation/1 -> Sum1/1
  Gain3/1 -> Transfer Fcn1/1
  Vd/1 -> Rate Transition9/1
  Add/1 -> Transfer Fcn/1
  Constant2/1 -> Add/1
  Transfer Fcn3/1 -> Add/3
  Constant1/1 -> Add/2
  Gain4/1 -> Sum8/1
  Transfer Fcn2/1 -> Add/4
  Sum7/1 -> Gain3/1
  Sum8/1 -> Sum7/2
  Transfer Fcn/1 -> Sum7/1
  Gain7/1 -> Sum8/2
  Transfer Fcn1/1 -> Gain7/1, Transfer Fcn2/1, Gain4/1, Saturation/1
  Gain1/1 -> Transfer Fcn3/1, Relational Operator1/1, Relational Operator/1
  Gain5/1 -> Relational Operator/2
  Gain6/1 -> Relational Operator1/2
  Relational Operator/1 -> Logical Operator/1
  Relational Operator1/1 -> Logical Operator/2
  Logical Operator/1 -> MO/1
  Constant4/1 -> Gain5/1, Gain6/1
  Rate Transition9/1 -> Gain1/1

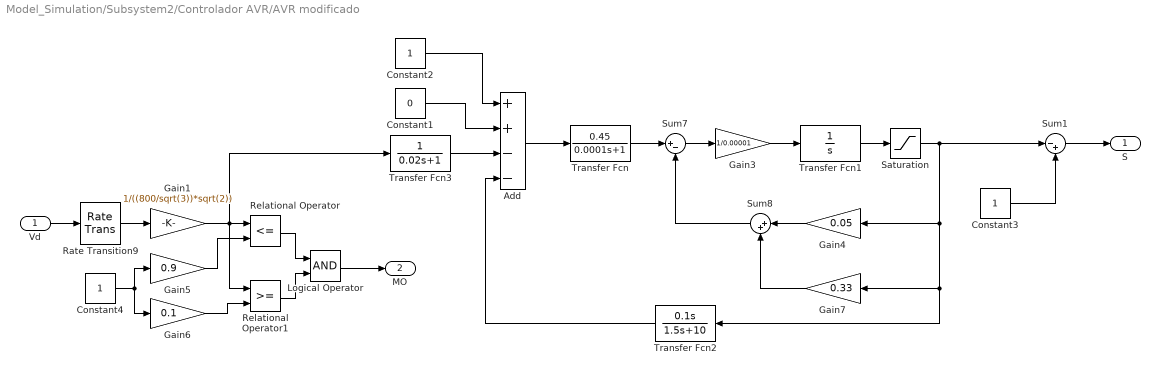
== system Model_Simulation/Subsystem2/Controlador AVR/AVR modificado ==
  Vd : Inport
  Add : Sum  Inputs=++--
  Constant1 : Constant  Value=0
  Constant2 : Constant
  Constant3 : Constant
  Constant4 : Constant
  Gain1 : Gain  Gain=1/((800/sqrt(3))*sqrt(2))
  Gain3 : Gain  Gain=1/0.00001
  Gain4 : Gain  Gain=0.05
  Gain5 : Gain  Gain=0.9
  Gain6 : Gain  Gain=0.1
  Gain7 : Gain  Gain=0.33
  Logical Operator : Logic  AllPortsSameDT=off  OutDataTypeStr=boolean
  Rate Transition9 : RateTransition  OutPortSampleTime=2e-6
  Relational Operator : RelationalOperator  Operator=<=  OutDataTypeStr=boolean
  Relational Operator1 : RelationalOperator  OutDataTypeStr=boolean
  Saturation : Saturate  UpperLimit=1  LowerLimit=0
  Sum1 : Sum  Inputs=|-+
  Sum7 : Sum  Inputs=|+-
  Sum8 : Sum  Inputs=|++
  Transfer Fcn : TransferFcn  Numerator=[0.45]  Denominator=[0.0001 1]
  Transfer Fcn1 : TransferFcn  Denominator=[1 0]
  Transfer Fcn2 : TransferFcn  Numerator=[0.1 0]  Denominator=[1.5 10]
  Transfer Fcn3 : TransferFcn  Denominator=[0.02 1]
  S : Outport
  MO : Outport  Port=2
  wires:
  Constant3/1 -> Sum1/2
  Sum1/1 -> S/1
  Saturation/1 -> Transfer Fcn2/1, Gain7/1, Gain4/1, Sum1/1
  Gain3/1 -> Transfer Fcn1/1
  Vd/1 -> Rate Transition9/1
  Add/1 -> Transfer Fcn/1
  Constant2/1 -> Add/1
  Transfer Fcn3/1 -> Add/3
  Constant1/1 -> Add/2
  Gain4/1 -> Sum8/1
  Transfer Fcn2/1 -> Add/4
  Sum7/1 -> Gain3/1
  Sum8/1 -> Sum7/2
  Transfer Fcn/1 -> Sum7/1
  Gain7/1 -> Sum8/2
  Gain1/1 -> Transfer Fcn3/1, Relational Operator1/1, Relational Operator/1
  Gain5/1 -> Relational Operator/2
  Gain6/1 -> Relational Operator1/2
  Relational Operator/1 -> Logical Operator/1
  Relational Operator1/1 -> Logical Operator/2
  Logical Operator/1 -> MO/1
  Constant4/1 -> Gain5/1, Gain6/1
  Rate Transition9/1 -> Gain1/1
  Transfer Fcn1/1 -> Saturation/1

== system Model_Simulation/Subsystem2/Controle do inversor/DQ0toABC ==
  note: dq2ABC
  Fase : Inport
  DQ0 : Inport  Port=2
  Demux1 : Demux  Outputs=3
  Fcn1 : Fcn  Commented=on  Expr=cos(u[1]-(2*pi/3))*u(2)+sin(u[1]-(2*pi/3))*u(3)+1*u(4)
  Fcn2 : Fcn  Commented=on  Expr=cos(u[1])*u(2)+sin(u[1])*u(3)+1*u(4)
  Fcn3 : Fcn  Commented=on  Expr=cos(u[1]+(2*pi/3))*u(2)+sin(u[1]+(2*pi/3))*u(3)+1*u(4)
  Gain1 : Gain  Gain=1/1500
  Gain2 : Gain  Gain=1/1500
  Gain3 : Gain  Gain=1/1500
  Transformada de Clarke alfa_beta_zero para abc : MATLAB Function  TreatAsAtomicUnit=on
  Transformada de Park dq0 para alfa_beta_zero : MATLAB Function  TreatAsAtomicUnit=on
  Va : Outport
  Vb : Outport  Port=2
  Vc : Outport  Port=3
  wires:
  Gain3/1 -> Vc/1
  Gain1/1 -> Vb/1
  Gain2/1 -> Va/1
  Transformada de Park dq0 para alfa_beta_zero/1(falfa) -> Transformada de Clarke alfa_beta_zero para abc/1(falfa)
  Transformada de Park dq0 para alfa_beta_zero/2(fbeta) -> Transformada de Clarke alfa_beta_zero para abc/2(fbeta)
  Transformada de Park dq0 para alfa_beta_zero/3(fzero) -> Transformada de Clarke alfa_beta_zero para abc/3(fzero)
  Fcn3/1 -> ?
  Fcn2/1 -> ?
  Fcn1/1 -> ?
  ? -> Fcn1/1
  ? -> Fcn3/1
  ? -> Fcn2/1
  Transformada de Clarke alfa_beta_zero para abc/2(fb) -> Gain1/1
  Transformada de Clarke alfa_beta_zero para abc/1(fa) -> Gain2/1
  Transformada de Clarke alfa_beta_zero para abc/3(fc) -> Gain3/1
  Demux1/1 -> Transformada de Park dq0 para alfa_beta_zero/1(fd)
  Demux1/2 -> Transformada de Park dq0 para alfa_beta_zero/2(fq)
  Demux1/3 -> Transformada de Park dq0 para alfa_beta_zero/3(f0)
  DQ0/1 -> Demux1/1
  Fase/1 -> Transformada de Park dq0 para alfa_beta_zero/4(theta)

== system Model_Simulation/Subsystem2/Conversor Boost Fotovoltaico/Arranjo 8 strings em paralelo com 43 módulos em série Vmp = 43 x 30,6 = 1315,8 V Imp = 8,32 x 7 = 58,24 A 76.632,192 W ==
  note: Vd=V_PV + Rs*I_PV
  S : Inport
  TempC : Inport  Port=2
  Add1 : Sum
  Diode Rsh : Subsystem
      mask Display:
      | plot(-75,-50,100,150, [-15 -15 43 -15 -15 -75],[50 8 50 92 50 50], ...
      |     [43 43],[8 94],[100 43], [50 50])
  Goto Tag Visibility : GotoTagVisibility  GotoTag=S_Sref
  Goto Tag Visibility1 : GotoTagVisibility  GotoTag=Vd
  Goto Tag Visibility2 : GotoTagVisibility  GotoTag=Tcell_K
  I Filter : spsPVarrayModel/No  VariantControl=Variant1
  IL : powerlib/Electrical Sources/Controlled Current Source  Initialize=on  Source_Type=AC  Amplitude=0  Phase=0  Frequency=0  Measurements=None
  IL ctrl : Subsystem
  I_PV : powerlib/Measurements/Current Measurement  PhasorSimulation=off  OutputType=Complex  PSBequivalent=0
  Product2 : Product  Inputs=**  RndMeth=Zero
  Rs_array : powerlib/Elements/Series RLC Branch  LConnTagsString=__new0  RConnTagsString=__new0  BranchType=R  Resistance=Rs*Nser/Npar  Inductance=1e-3  SetiL0=off  InitialCurrent=0  Capacitance=1e-6  Setx0=off  InitialVoltage=0  Measurements=None
  Rs_array_ : Constant  Value=Rs*Nser/Npar
  Rsh_array For 0.05*Sref : powerlib/Elements/Series RLC Branch  LConnTagsString=__new0  RConnTagsString=__new0  BranchType=R  Resistance=Rsh_array5pc  Inductance=1e-3  SetiL0=off  InitialCurrent=0  Capacitance=1e-6  Setx0=off  InitialVoltage=0  Measurements=None
  V Filter : spsPVarrayModel/No  VariantControl=Variant1
  V_PV : powerlib/Measurements/Voltage Measurement  PhasorSimulation=off  OutputType=Complex  PSBequivalent=0
  + : PMIOPort  Port=1  Side=Right
  - : PMIOPort  Port=2  Side=Right
  tag scope: Vd=scoped
  wires:
  TempC/1 -> IL ctrl/1(Temperature)  "Temperature (deg C)"
  S/1 -> IL ctrl/2(Irradiance)  "Irradiance (W/m2)"
  Add1/1 -> [Vd]  "Vd"
  I_PV/1 -> I Filter/1  "I_PV"
  Product2/1 -> Add1/2
  Rs_array_/1 -> Product2/2
  IL ctrl/1(IL) -> IL/1
  V_PV/1 -> V Filter/1
  I Filter/1 -> Product2/1  "I_PV"
  V Filter/1 -> Add1/1  "V_PV"
  connections:
  +/RConn1 -- I_PV/RConn1 -- V_PV/LConn1
  Diode Rsh/LConn1 -- Rs_array/LConn1 -- Rsh_array For 0.05*Sref/LConn1 -- IL/RConn1
  V_PV/LConn2 -- -/RConn1 -- Rsh_array For 0.05*Sref/RConn1 -- Diode Rsh/RConn1 -- IL/LConn1
  Rs_array/RConn1 -- I_PV/LConn1

== system Model_Simulation/Subsystem2/Conversor Boost Fotovoltaico/Signal Builder2 ==
  Demux : Demux  Tag=STV Demux  Outputs=1
  FromWs : FromWorkspace  Tag=STV FromWs  VariableName=tuvar  SampleTime=0
      SigBuilderData=|
      | common.afterFinalStr = 'Extrapolate'
      | common.sampleTime = 0
      | dataSet.timeRange = [0 10]
      | dataSet.name = 'Group 1'
      | sbobj.Groups.Name = 'Group 1'
      | sbobj.Groups.Signals.Name = 'Signal 2'
      | sbobj.Groups.Signals.XData = [0 0.2 0.2 0.6 0.8 1.6 1.6 2 2 5 5 6 6 7 7 8 8 9 9 10]
      | sbobj.Groups.Signals.YData = [1000 1000 500 500 1000 1000 200 200 1000 1000 0 0 1000 1000 0 0 1000 1000 0 0]
  Signal 2 : Outport  Tag=STV Outport
  wires:
  Demux/1 -> Signal 2/1
  FromWs/1 -> Demux/1

== system Model_Simulation/Subsystem2/Conversor Boost Fotovoltaico1/Arranjo 8 strings em paralelo com 43 módulos em série Vmp = 43 x 30,6 = 1315,8 V Imp = 8,32 x 7 = 58,24 A 76.632,192 W ==
  note: Vd=V_PV + Rs*I_PV
  S : Inport
  TempC : Inport  Port=2
  Add1 : Sum
  Diode Rsh : Subsystem
      mask Display:
      | plot(-75,-50,100,150, [-15 -15 43 -15 -15 -75],[50 8 50 92 50 50], ...
      |     [43 43],[8 94],[100 43], [50 50])
  Goto Tag Visibility : GotoTagVisibility  GotoTag=S_Sref
  Goto Tag Visibility1 : GotoTagVisibility  GotoTag=Vd
  Goto Tag Visibility2 : GotoTagVisibility  GotoTag=Tcell_K
  I Filter : spsPVarrayModel/No  VariantControl=Variant1
  IL : powerlib/Electrical Sources/Controlled Current Source  Initialize=on  Source_Type=AC  Amplitude=0  Phase=0  Frequency=0  Measurements=None
  IL ctrl : Subsystem
  I_PV : powerlib/Measurements/Current Measurement  PhasorSimulation=off  OutputType=Complex  PSBequivalent=0
  Product2 : Product  Inputs=**  RndMeth=Zero
  Rs_array : powerlib/Elements/Series RLC Branch  LConnTagsString=__new0  RConnTagsString=__new0  BranchType=R  Resistance=Rs*Nser/Npar  Inductance=1e-3  SetiL0=off  InitialCurrent=0  Capacitance=1e-6  Setx0=off  InitialVoltage=0  Measurements=None
  Rs_array_ : Constant  Value=Rs*Nser/Npar
  Rsh_array For 0.05*Sref : powerlib/Elements/Series RLC Branch  LConnTagsString=__new0  RConnTagsString=__new0  BranchType=R  Resistance=Rsh_array5pc  Inductance=1e-3  SetiL0=off  InitialCurrent=0  Capacitance=1e-6  Setx0=off  InitialVoltage=0  Measurements=None
  V Filter : spsPVarrayModel/No  VariantControl=Variant1
  V_PV : powerlib/Measurements/Voltage Measurement  PhasorSimulation=off  OutputType=Complex  PSBequivalent=0
  + : PMIOPort  Port=1  Side=Right
  - : PMIOPort  Port=2  Side=Right
  tag scope: Vd=scoped
  wires:
  V Filter/1 -> Add1/1  "V_PV"
  I Filter/1 -> Product2/1  "I_PV"
  V_PV/1 -> V Filter/1
  IL ctrl/1(IL) -> IL/1
  Rs_array_/1 -> Product2/2
  Product2/1 -> Add1/2
  I_PV/1 -> I Filter/1  "I_PV"
  Add1/1 -> [Vd]  "Vd"
  S/1 -> IL ctrl/2(Irradiance)  "Irradiance (W/m2)"
  TempC/1 -> IL ctrl/1(Temperature)  "Temperature (deg C)"
  connections:
  Rs_array/RConn1 -- I_PV/LConn1
  IL/LConn1 -- Diode Rsh/RConn1 -- Rsh_array For 0.05*Sref/RConn1 -- -/RConn1 -- V_PV/LConn2
  IL/RConn1 -- Rsh_array For 0.05*Sref/LConn1 -- Rs_array/LConn1 -- Diode Rsh/LConn1
  V_PV/LConn1 -- I_PV/RConn1 -- +/RConn1

== system Model_Simulation/Subsystem2/Conversor Boost Fotovoltaico1/Signal Builder2 ==
  Demux : Demux  Tag=STV Demux  Outputs=1
  FromWs : FromWorkspace  Tag=STV FromWs  VariableName=tuvar  SampleTime=0
      SigBuilderData=|
      | common.afterFinalStr = 'Extrapolate'
      | common.sampleTime = 0
      | dataSet.timeRange = [0 10]
      | dataSet.name = 'Group 1'
      | sbobj.Groups.Name = 'Group 1'
      | sbobj.Groups.Signals.Name = 'Signal 2'
      | sbobj.Groups.Signals.XData = [0 0.2 0.2 0.6 0.8 1.6 1.6 2 2 5 5 6 6 7 7 8 8 9 9 10]
      | sbobj.Groups.Signals.YData = [1000 1000 500 500 1000 1000 200 200 1000 1000 0 0 1000 1000 0 0 1000 1000 0 0]
  Signal 2 : Outport  Tag=STV Outport
  wires:
  FromWs/1 -> Demux/1
  Demux/1 -> Signal 2/1

== system Model_Simulation/Subsystem2/Conversor Boost Fotovoltaico2/Arranjo 8 strings em paralelo com 43 módulos em série Vmp = 43 x 30,6 = 1315,8 V Imp = 8,32 x 7 = 58,24 A 76.632,192 W ==
  note: Vd=V_PV + Rs*I_PV
  S : Inport
  TempC : Inport  Port=2
  Add1 : Sum
  Diode Rsh : Subsystem
      mask Display:
      | plot(-75,-50,100,150, [-15 -15 43 -15 -15 -75],[50 8 50 92 50 50], ...
      |     [43 43],[8 94],[100 43], [50 50])
  Goto Tag Visibility : GotoTagVisibility  GotoTag=S_Sref
  Goto Tag Visibility1 : GotoTagVisibility  GotoTag=Vd
  Goto Tag Visibility2 : GotoTagVisibility  GotoTag=Tcell_K
  I Filter : spsPVarrayModel/No  VariantControl=Variant1
  IL : powerlib/Electrical Sources/Controlled Current Source  Initialize=on  Source_Type=AC  Amplitude=0  Phase=0  Frequency=0  Measurements=None
  IL ctrl : Subsystem
  I_PV : powerlib/Measurements/Current Measurement  PhasorSimulation=off  OutputType=Complex  PSBequivalent=0
  Product2 : Product  Inputs=**  RndMeth=Zero
  Rs_array : powerlib/Elements/Series RLC Branch  LConnTagsString=__new0  RConnTagsString=__new0  BranchType=R  Resistance=Rs*Nser/Npar  Inductance=1e-3  SetiL0=off  InitialCurrent=0  Capacitance=1e-6  Setx0=off  InitialVoltage=0  Measurements=None
  Rs_array_ : Constant  Value=Rs*Nser/Npar
  Rsh_array For 0.05*Sref : powerlib/Elements/Series RLC Branch  LConnTagsString=__new0  RConnTagsString=__new0  BranchType=R  Resistance=Rsh_array5pc  Inductance=1e-3  SetiL0=off  InitialCurrent=0  Capacitance=1e-6  Setx0=off  InitialVoltage=0  Measurements=None
  V Filter : spsPVarrayModel/No  VariantControl=Variant1
  V_PV : powerlib/Measurements/Voltage Measurement  PhasorSimulation=off  OutputType=Complex  PSBequivalent=0
  + : PMIOPort  Port=1  Side=Right
  - : PMIOPort  Port=2  Side=Right
  tag scope: Vd=scoped
  wires:
  TempC/1 -> IL ctrl/1(Temperature)  "Temperature (deg C)"
  S/1 -> IL ctrl/2(Irradiance)  "Irradiance (W/m2)"
  Add1/1 -> [Vd]  "Vd"
  I_PV/1 -> I Filter/1  "I_PV"
  Product2/1 -> Add1/2
  Rs_array_/1 -> Product2/2
  IL ctrl/1(IL) -> IL/1
  V_PV/1 -> V Filter/1
  I Filter/1 -> Product2/1  "I_PV"
  V Filter/1 -> Add1/1  "V_PV"
  connections:
  +/RConn1 -- I_PV/RConn1 -- V_PV/LConn1
  Diode Rsh/LConn1 -- Rs_array/LConn1 -- Rsh_array For 0.05*Sref/LConn1 -- IL/RConn1
  V_PV/LConn2 -- -/RConn1 -- Rsh_array For 0.05*Sref/RConn1 -- Diode Rsh/RConn1 -- IL/LConn1
  Rs_array/RConn1 -- I_PV/LConn1

== system Model_Simulation/Subsystem2/Conversor Boost Fotovoltaico2/Signal Builder2 ==
  Demux : Demux  Tag=STV Demux  Outputs=1
  FromWs : FromWorkspace  Tag=STV FromWs  VariableName=tuvar  SampleTime=0
      SigBuilderData=|
      | common.afterFinalStr = 'Extrapolate'
      | common.sampleTime = 0
      | dataSet.timeRange = [0 10]
      | dataSet.name = 'Group 1'
      | sbobj.Groups.Name = 'Group 1'
      | sbobj.Groups.Signals.Name = 'Signal 2'
      | sbobj.Groups.Signals.XData = [0 0.2 0.2 0.6 0.8 1.6 1.6 2 2 5 5 6 6 7 7 8 8 9 9 10]
      | sbobj.Groups.Signals.YData = [1000 1000 500 500 1000 1000 200 200 1000 1000 0 0 1000 1000 0 0 1000 1000 0 0]
  Signal 2 : Outport  Tag=STV Outport
  wires:
  Demux/1 -> Signal 2/1
  FromWs/1 -> Demux/1

== system Model_Simulation/Subsystem2/DDSRF-PLL /Subsystem ==
  Fase : Inport
  Alpha : Inport  Port=2
  Beta : Inport  Port=3
  Gain : Gain  Gain=-1
  Product{,1..3} (4 alike) : Product
  Sum : Sum  Inputs=|++
  Sum1 : Sum  Inputs=|++
  Trigonometric Function : Trigonometry
  Trigonometric Function1 : Trigonometry  Operator=cos
  Trigonometric Function2 : Trigonometry
  Trigonometric Function3 : Trigonometry  Operator=cos
  Vd+ : Outport
  Vq+ : Outport  Port=2
  wires:
  Alpha/1 -> Gain/1, Product1/2
  Trigonometric Function/1 -> Product/1
  Beta/1 -> Product3/2, Product/2
  Fase/1 -> Trigonometric Function3/1, Trigonometric Function2/1, Trigonometric Function1/1, Trigonometric Function/1
  Product/1 -> Sum/1
  Product1/1 -> Sum/2
  Trigonometric Function1/1 -> Product1/1
  Sum/1 -> Vd+/1
  Trigonometric Function2/1 -> Product2/1
  Product2/1 -> Sum1/1
  Sum1/1 -> Vq+/1
  Gain/1 -> Product2/2
  Trigonometric Function3/1 -> Product3/1
  Product3/1 -> Sum1/2

== system Model_Simulation/Subsystem2/DDSRF-PLL /Subsystem1 ==
  Fase : Inport
  Alpha : Inport  Port=2
  Beta : Inport  Port=3
  Gain1 : Gain  Gain=-1
  Product{,1..3} (4 alike) : Product
  Sum : Sum  Inputs=|++
  Sum1 : Sum  Inputs=|++
  Trigonometric Function : Trigonometry
  Trigonometric Function1 : Trigonometry  Operator=cos
  Trigonometric Function2 : Trigonometry
  Trigonometric Function3 : Trigonometry  Operator=cos
  Vd- : Outport
  Vq- : Outport  Port=2
  wires:
  Product3/1 -> Sum1/2
  Trigonometric Function3/1 -> Product3/1
  Alpha/1 -> Product2/2, Product1/2
  Sum1/1 -> Vq-/1
  Product2/1 -> Sum1/1
  Trigonometric Function2/1 -> Product2/1
  Sum/1 -> Vd-/1
  Trigonometric Function1/1 -> Product1/1
  Product1/1 -> Sum/2
  Product/1 -> Sum/1
  Fase/1 -> Trigonometric Function1/1, Trigonometric Function2/1, Trigonometric Function3/1, Trigonometric Function/1
  Beta/1 -> Gain1/1, Product3/2
  Trigonometric Function/1 -> Product/1
  Gain1/1 -> Product/2

== system Model_Simulation/Subsystem2/DDSRF-PLL /Subsystem2 ==
  Vd+ : Inport
  Vq+ : Inport  Port=2
  Vd- : Inport  Port=3
  Vq- : Inport  Port=4
  fase : Inport  Port=5
  Gain : Gain  Gain=2
  Product{,1..3} (4 alike) : Product
  Sum1 : Sum  Inputs=|+-
  Sum2 : Sum  Inputs=|+-
  Sum3 : Sum  Inputs=|+-
  Sum4 : Sum  Inputs=|++
  Trigonometric Function1 : Trigonometry  Operator=cos
  Trigonometric Function2 : Trigonometry
  Vd*+ : Outport
  Vq*+ : Outport  Port=2
  wires:
  Sum1/1 -> Vq*+/1
  Sum3/1 -> Vd*+/1
  Vd+/1 -> Sum2/1
  Vd-/1 -> Product3/2, Product/1
  Product/1 -> Sum2/2
  Trigonometric Function1/1 -> Product2/2, Product/2
  fase/1 -> Gain/1
  Gain/1 -> Trigonometric Function1/1, Trigonometric Function2/1
  Sum2/1 -> Sum3/1
  Product1/1 -> Sum3/2
  Vq-/1 -> Product2/1, Product1/1
  Product2/1 -> Sum1/2
  Trigonometric Function2/1 -> Product1/2, Product3/1
  Vq+/1 -> Sum4/1
  Product3/1 -> Sum4/2
  Sum4/1 -> Sum1/1

== system Model_Simulation/Subsystem2/DDSRF-PLL /Subsystem3 ==
  Vd- : Inport
  Vq- : Inport  Port=2
  Vd+ : Inport  Port=3
  Vq+ : Inport  Port=4
  fase : Inport  Port=5
  Gain : Gain  Gain=-2
  Product{,1..3} (4 alike) : Product
  Sum1 : Sum  Inputs=|+-
  Sum2 : Sum  Inputs=|+-
  Sum3 : Sum  Inputs=|+-
  Sum4 : Sum  Inputs=|++
  Trigonometric Function1 : Trigonometry  Operator=cos
  Trigonometric Function2 : Trigonometry
  Vd*- : Outport
  Vq*- : Outport  Port=2
  wires:
  Sum4/1 -> Sum1/1
  Product3/1 -> Sum4/2
  Vq-/1 -> Sum4/1
  Trigonometric Function2/1 -> Product3/1, Product1/2
  Product2/1 -> Sum1/2
  Vq+/1 -> Product1/1, Product2/1
  Product1/1 -> Sum3/2
  Sum2/1 -> Sum3/1
  Gain/1 -> Trigonometric Function2/1, Trigonometric Function1/1
  fase/1 -> Gain/1
  Trigonometric Function1/1 -> Product/2, Product2/2
  Product/1 -> Sum2/2
  Vd+/1 -> Product/1, Product3/2
  Vd-/1 -> Sum2/1
  Sum3/1 -> Vd*-/1
  Sum1/1 -> Vq*-/1

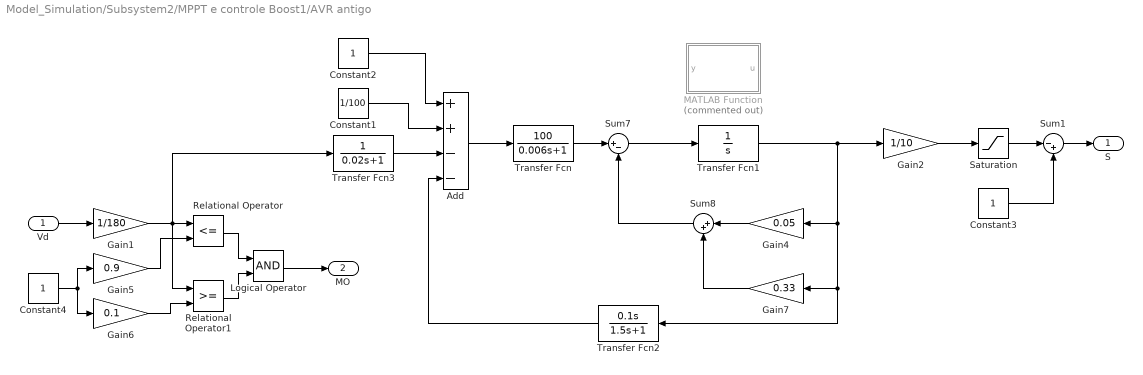
== system Model_Simulation/Subsystem2/MPPT e controle Boost1/AVR antigo ==
  Vd : Inport
  Add : Sum  Inputs=++--
  Constant1 : Constant  Value=1/100
  Constant2 : Constant
  Constant3 : Constant
  Constant4 : Constant
  Gain1 : Gain  Gain=1/180
  Gain2 : Gain  Gain=1/10
  Gain4 : Gain  Gain=0.05
  Gain5 : Gain  Gain=0.9
  Gain6 : Gain  Gain=0.1
  Gain7 : Gain  Gain=0.33
  Logical Operator : Logic  AllPortsSameDT=off  OutDataTypeStr=boolean
  MATLAB Function : MATLAB Function  Commented=on  TreatAsAtomicUnit=on
  Relational Operator : RelationalOperator  Operator=<=  OutDataTypeStr=boolean
  Relational Operator1 : RelationalOperator  OutDataTypeStr=boolean
  Saturation : Saturate  UpperLimit=1  LowerLimit=0
  Sum1 : Sum  Inputs=|-+
  Sum7 : Sum  Inputs=|+-
  Sum8 : Sum  Inputs=|++
  Transfer Fcn : TransferFcn  Numerator=[100]  Denominator=[0.006 1]
  Transfer Fcn1 : TransferFcn  Denominator=[1 0]
  Transfer Fcn2 : TransferFcn  Numerator=[0.1 0]  Denominator=[1.5 1]
  Transfer Fcn3 : TransferFcn  Denominator=[0.02 1]
  S : Outport
  MO : Outport  Port=2
  wires:
  Constant3/1 -> Sum1/2
  Sum1/1 -> S/1
  Saturation/1 -> Sum1/1
  Constant4/1 -> Gain6/1, Gain5/1
  Transfer Fcn1/1 -> Gain4/1, Transfer Fcn2/1, Gain7/1, Gain2/1
  Logical Operator/1 -> MO/1
  Relational Operator1/1 -> Logical Operator/2
  Relational Operator/1 -> Logical Operator/1
  Gain6/1 -> Relational Operator1/2
  Gain5/1 -> Relational Operator/2
  Gain1/1 -> Relational Operator/1, Relational Operator1/1, Transfer Fcn3/1
  Gain2/1 -> Saturation/1
  Gain7/1 -> Sum8/2
  Transfer Fcn/1 -> Sum7/1
  Sum8/1 -> Sum7/2
  Sum7/1 -> Transfer Fcn1/1
  Transfer Fcn2/1 -> Add/4
  Gain4/1 -> Sum8/1
  Constant1/1 -> Add/2
  Transfer Fcn3/1 -> Add/3
  Constant2/1 -> Add/1
  Add/1 -> Transfer Fcn/1
  Vd/1 -> Gain1/1

== system Model_Simulation/Subsystem2/Arranjo 21 strings em paralelo com 43 módulos em série Vmp = 43 x 30,6 = 1315,8 V Imp = 8,32 x 21 = 174,72 A 229.896,576 W/Diode Rsh/Subsystem ==
  note: exp((EgRef/(k1*Tref_K))-(E_g/(k1*Tcell_K)))
  Tcell_K : Inport
  E_g : Inport  Port=2
  Add : Sum  Inputs=+-
  EgRef : Constant  Value=EgRef/(k1*Tref_K)
  Math Function : Math  SaturateOnIntegerOverflow=on
  Product : Product  Inputs=*/
  k1 : Gain  Gain=k1
  exp : Outport
  wires:
  Math Function/1 -> exp/1
  Add/1 -> Math Function/1
  Product/1 -> Add/2
  k1/1 -> Product/2
  Tcell_K/1 -> k1/1
  E_g/1 -> Product/1
  EgRef/1 -> Add/1
